simulink model "model1"  (R2024b)
settings: Solver=ode45  StartTime=0.0  StopTime=20  MaxStep=inf  RelTol=1e-6
PreLoadFcn:
  | % referenced workspace parameters
  | 
  | % tunable
  | mu = 1;
  | dx2min = -inf;
  | dx2max = inf;
  | x1IC = 2;
  | 
  | % non-tunable
  | uST = 1;
settings Model: Creator=mural  LastModifiedBy=murali
settings DataIOCC: SaveOutput=off  DSMLogging=off  SaveTime=off
settings OptimizationCC: ReuseModelBlockBuffer=off
settings DebuggingCC: UnconnectedInputMsg=warning  UnconnectedOutputMsg=warning  UnconnectedLineMsg=warning
settings ModelReferenceCC: EnableRefExpFcnMdlSchedulingChecks=on
settings RTWCC: GPUComputeCapability=3.5  DLArmComputeVersion=19.05

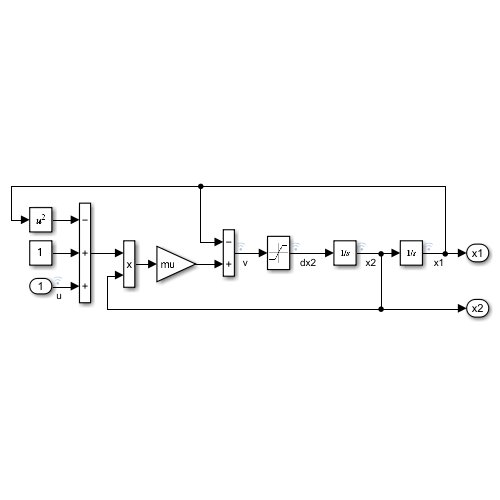
[thumbnail: Simulink's stored preview of the top-level diagram]
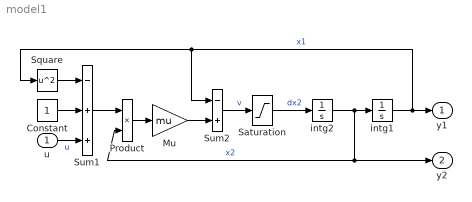
== system model1 ==
  u : Inport  SampleTime=uST  Interpolate=off
  Constant : Constant
  Mu : Gain  Gain=mu  SaturateOnIntegerOverflow=on  OutDataTypeStr=Inherit: Same as input  ParamDataTypeStr=Inherit: Same as input
  Product : Product  InputSameDT=on  RndMeth=Zero  SaturateOnIntegerOverflow=on  OutDataTypeStr=Inherit: Same as first input
  Saturation : Saturate  UpperLimit=dx2max  LowerLimit=dx2min
  Square : Math  Operator=square
  Sum1 : Sum  Inputs=-++  InputSameDT=on  SaturateOnIntegerOverflow=on  OutDataTypeStr=Inherit: Same as first input
  Sum2 : Sum  Inputs=-+  InputSameDT=on  SaturateOnIntegerOverflow=on  OutDataTypeStr=Inherit: Same as first input
  intg1 : Integrator  InitialCondition=x1IC
  intg2 : Integrator
  y1 : Outport  InitialOutput=0  VectorParamsAs1DForOutWhenUnconnected=off
  y2 : Outport  Port=2  InitialOutput=0  VectorParamsAs1DForOutWhenUnconnected=off
  wires:
  Saturation/1 -> intg2/1  "dx2"
  u/1 -> Sum1/3  "u"
  Sum1/1 -> Product/1
  Constant/1 -> Sum1/2
  Square/1 -> Sum1/1
  Mu/1 -> Sum2/2
  Product/1 -> Mu/1
  intg1/1 -> Square/1, Sum2/1, y1/1  "x1"
  intg2/1 -> y2/1, Product/2, intg1/1  "x2"
  Sum2/1 -> Saturation/1  "v"
